simulink model "BusCreatorEnum_nonvirtual"  (R2017b)
settings: Solver=FixedStepDiscrete  StartTime=0.0  StopTime=10.0  FixedStep=0.200000  RelTol=1e-3
PreLoadFcn:
  | % Bus object: subBus
  | clear elems;
  | elems(1) = Simulink.BusElement;
  | elems(1).Name = 'chirp';
  | elems(1).Dimensions = 1;
  | elems(1).DimensionsMode = 'Fixed';
  | elems(1).DataType = 'Enum: Days';
  | elems(1).SampleTime = -1;
  | elems(1).Complexity = 'real';
  | elems(1).Min = [];
  | elems(1).Max = [];
  | elems(1).DocUnits = '';
  | elems(1).Description = '';
  | 
  | elems(2) = Simulink.BusElement;
  | elems(2).Name = 'sine';
  | elems(2).Dimensions = 3;
  | elems(2).DimensionsMode = 'Fixed';
  | elems(2).DataType = 'int32';
  | elems(2).SampleTime = -1;
  | elems(2).Complexity = 'real';
  | elems(2).Min = [];
  | elems(2).Max = [];
  | elems(2).DocUnits = '';
  | elems(2).Description = '';
  | 
  | subBus = Simulink.Bus;
  | subBus.HeaderFile = '';
  | subBus.Description = '';
  | subBus.DataScope = 'Auto';
  | subBus.Alignment = -1;
  | subBus.Elements = elems;
  | clear elems;
  | assignin('base','subBus', subBus);
  | 
  | % Bus object: topBus
  | clear elems;
  | elems(1) = Simulink.BusElement;
  | elems(1).Name = 'subSignal';
  | elems(1).Dimensions = 1;
  | elems(1).DimensionsMode = 'Fixed';
  | elems(1).DataType = 'Bus: subBus';
  | elems(1).SampleTime = -1;
  | elems(1).Complexity = 'real';
  | elems(1).Min = [];
  | elems(1).Max = [];
  | elems(1).DocUnits = '';
  | elems(1).Description = '';
  | 
  | elems(2) = Simulink.BusElement;
  | elems(2).Name = 'step';
  | elems(2).Dimensions = 4;
  | elems(2).DimensionsMode = 'Fixed';
  | elems(2).DataType = 'boolean';
  | elems(2).SampleTime = -1;
  | elems(2).Complexity = 'real';
  | elems(2).Min = [];
  | elems(2).Max = [];
  | elems(2).DocUnits = '';
  | elems(2).Description = '';
  | 
  | topBus = Simulink.Bus;
  | topBus.HeaderFile = '';
  | topBus.Description = '';
  | topBus.DataScope = 'Auto';
  | topBus.Alignment = -1;
  | topBus.Elements = elems;
  | clear elems;
  | assignin('base','topBus', topBus);
undefined symbols (not defined in the file): Days
libraries: simulink x1
settings Model: Creator=The MathWorks, Inc.  LastModifiedBy=hbourbou
settings OptimizationCC: LifeSpan=inf
settings DebuggingCC: SFExecutionAtInitializationDiag=none
settings HardwareCC: ProdBitPerSizeT=32  ProdBitPerPtrDiffT=32  ProdWordSize=32  ProdHWDeviceType=Specified
settings CodeAppCC: StateflowObjectComments=on
settings ConfigComp: CovMetricSettings=dswe

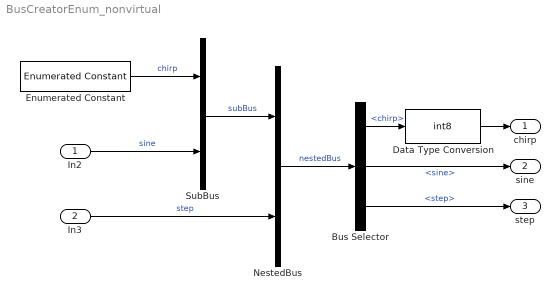
== system BusCreatorEnum_nonvirtual ==
  In2 : Inport  OutDataTypeStr=int32  PortDimensions=3
  In3 : Inport  Port=2  OutDataTypeStr=boolean  PortDimensions=4
  Bus Selector : BusSelector  OutputSignals=subBus.chirp,subBus.sine,step
  Data Type Conversion : DataTypeConversion  OutDataTypeStr=int8
  Enumerated Constant : simulink/Sources/Enumerated Constant  OutDataTypeStr=Enum: Days  Value=Days.Sunday  SampleTime=inf
      settings: SourceProductName=Simulink
  NestedBus : BusCreator  Inputs=2  OutDataTypeStr=Bus: topBus  NonVirtualBus=on
      settings: AttributesFormatString=NestedBus
  SubBus : BusCreator  Inputs=2  OutDataTypeStr=Bus: subBus  NonVirtualBus=on
      settings: AttributesFormatString=SubBus
  chirp : Outport
  sine : Outport  Port=2
  step : Outport  Port=3
  wires:
  Enumerated Constant/1 -> SubBus/1  "chirp"
  SubBus/1 -> NestedBus/1  "subBus"
  In2/1 -> SubBus/2  "sine"
  In3/1 -> NestedBus/2  "step"
  NestedBus/1 -> Bus Selector/1  "nestedBus"
  Bus Selector/1 -> Data Type Conversion/1  "<chirp>"
  Bus Selector/2 -> sine/1  "<sine>"
  Bus Selector/3 -> step/1  "<step>"
  Data Type Conversion/1 -> chirp/1
